simulink model "non_linear_sys_2"  (R2021b)
settings: Solver=FixedStepAuto  StartTime=0.0  StopTime=tfinal  FixedStep=dt  RelTol=1e-3
values from neighbouring files (symbols this model uses):
  dt = 1e-3    (= 0.001)    [data.m]
  g = 9.81    [data.m]
  IC = [0.0 0.0]    [data.m]    (also in postproc2.m)
  Jb = 2/5 * mb * rb^2    (= 4.24e-05)    [data.m]
  Lx = 0.143    [data.m]    (also in robust.m = Rx*M*Gx)
  Ly = 0.184    [data.m]    (also in robust.m = Rx*M*Gy)
  mb = 0.265    [data.m]    (also in robust.m = ureal('mb',mb,'Percentage',50))
  PID_sim = PID(PID_idx(ii))    [postproc2.m]
  rb = 0.02    [data.m]    (also in robust.m = ureal('rb',rb,'Percentage',20))
  rm = 0.025    [data.m]
undefined symbols (not defined in the file or in its folder): ref
libraries: simulink x6, slpidlib x2
settings Model: Creator=Daniele Oranges  LastModifiedBy=Daniele Oranges

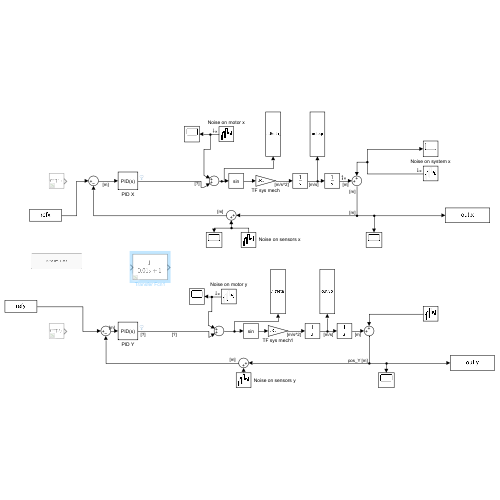
[thumbnail: Simulink's stored preview of the top-level diagram]
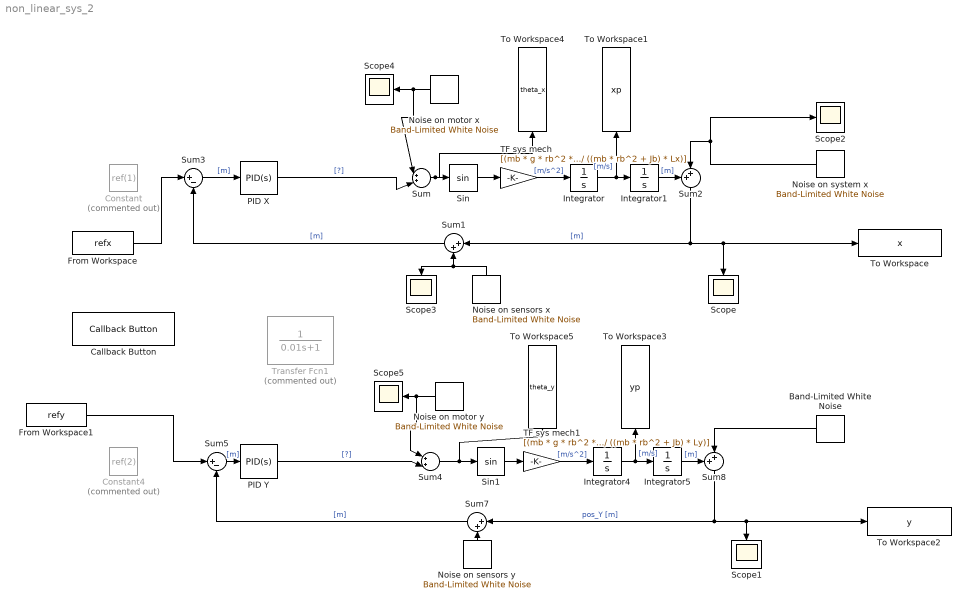
== system non_linear_sys_2 ==
  Band-Limited White Noise : simulink/Sources/Band-Limited White Noise  Cov=N.system  Ts=dt  seed=[23341]
  Callback Button : CallbackButton  ButtonText=Initialize Data
      settings: ClickFcn=|
      | clear
      | data
  Constant : Constant  Commented=on  Value=ref(1)
  Constant4 : Constant  Commented=on  Value=ref(2)
  From Workspace : FromWorkspace  VariableName=refx
  From Workspace1 : FromWorkspace  VariableName=refy
  Integrator : Integrator  InitialCondition=IC.velocity(1)
  Integrator1 : Integrator  InitialCondition=IC.position(1)
  Integrator4 : Integrator  InitialCondition=IC.velocity(2)
  Integrator5 : Integrator  InitialCondition=IC.position(2)
  Noise on motor x : simulink/Sources/Band-Limited White Noise  Cov=N.tension  Ts=dt  seed=[23341]
  Noise on motor y : simulink/Sources/Band-Limited White Noise  Cov=N.tension  Ts=dt  seed=[23341]
  Noise on sensors x : simulink/Sources/Band-Limited White Noise  Cov=N.sensor  Ts=dt  seed=[23341]
  Noise on sensors y : simulink/Sources/Band-Limited White Noise  Cov=N.sensor  Ts=dt  seed=[23341]
  Noise on system x : simulink/Sources/Band-Limited White Noise  Cov=N.system  Ts=dt  seed=[23341]
  PID X : slpidlib/PID Controller  Controller=PID  Form=Parallel  TimeDomain=Continuous-time  UseExternalTs=off  SampleTime=-1  IntegratorMethod=Forward Euler  FilterMethod=Forward Euler  ControllerParametersSource=internal  P=PID_sim.Kp  I=PID_sim.Ki  D=PID_sim.Kd  UseFilter=on  N=PID_sim.filter  TunerSelectOption=Transfer Function Based (PID Tuner App)  InitialConditionSource=internal  InitialConditionForIntegrator=0  InitialConditionForFilter=0  DifferentiatorICPrevScaledInput=0  ExternalReset=none  TrackingMode=off  Kt=1  LimitOutput=off  SatLimitsSource=internal  UpperSaturationLimit=inf  LowerSaturationLimit=-inf  LinearizeAsGain=on  AntiWindupMode=none  Kb=1  POutMin=[]  POutMax=[]  IOutMin=[]  IOutMax=[]  DOutMin=[]  DOutMax=[]  NOutMin=[]  NOutMax=[]  SumOutMin=[]  SumOutMax=[]  SaturationOutMin=[]  SaturationOutMax=[]  PParamMin=[]  PParamMax=[]  IParamMin=[]  IParamMax=[]  DParamMin=[]  DParamMax=[]  NParamMin=[]  NParamMax=[]  KbParamMin=[]  KbParamMax=[]  KtParamMin=[]  KtParamMax=[]  KbOutMin=[]  KbOutMax=[]  KtOutMin=[]  KtOutMax=[]  IntegratorOutMin=[]  IntegratorOutMax=[]  FilterOutMin=[]  FilterOutMax=[]  SumI1OutMin=[]  SumI1OutMax=[]  SumI2OutMin=[]  SumI2OutMax=[]  SumI3OutMin=[]  SumI3OutMax=[]  SumI4OutMin=[]  SumI4OutMax=[]  SumDOutMin=[]  SumDOutMax=[]  DifferentiatorOutMin=[]  DifferentiatorOutMax=[]  FilterDiffOutCoefMin=[]  FilterDiffOutCoefMax=[]  ReciprocalOutMin=[]  ReciprocalOutMax=[]  SumDenOutMin=[]  SumDenOutMax=[]  SumNumOutMin=[]  SumNumOutMax=[]  DivideOutMin=[]  DivideOutMax=[]  UdiffTsProdOutMin=[]  UdiffTsProdOutMax=[]  NTsProdOutMin=[]  NTsProdOutMax=[]  UintegralTsProdOutMin=[]  UintegralTsProdOutMax=[]  UngainTsProdOutMin=[]  UngainTsProdOutMax=[]  IntegratorContinuousStateAttributes=''  IntegratorStateMustResolveToSignalObject=off  IntegratorRTWStateStorageClass=Auto  FilterContinuousStateAttributes=''  FilterStateMustResolveToSignalObject=off  FilterRTWStateStorageClass=Auto  ParallelPVariant=InternalParameters  IdealPVariant=Disabled  IVariant=InternalParameters  DVariant=InternalParameters  IntegratorVariant=Continuous  SatVariant=Disabled  AWVariant=Passthrough  PCopyVariant=Disabled  TRVariant=Disabled  FdbkBlocksVariant=Forward  IdealPFdbkVariant=Disabled  SatFdbkVariant=Disabled  DerivativeFilterVariant=ContFilter  NVariant=InternalParameters  NCopyVariant=Disabled  FilterICVariant=InternalICsFilter  IntegratorICVariant=InternalICs  ExternalResetVariant=Disabled  TRSumVariant=Passthrough  SumFdbkVariant=Disabled  SumVariant=Sum_PID  TsampFilterVariant=InternalTs  TsampNgainVariant=Passthrough  TsampIntegralVariant=Passthrough  ExternalSaturationOutDataTypeStr=Inherit: Same as second input
  PID Y : slpidlib/PID Controller  Controller=PID  Form=Parallel  TimeDomain=Continuous-time  UseExternalTs=off  SampleTime=-1  IntegratorMethod=Forward Euler  FilterMethod=Forward Euler  ControllerParametersSource=internal  P=PID_sim.Kp  I=PID_sim.Ki  D=PID_sim.Kd  UseFilter=on  N=PID_sim.filter  TunerSelectOption=Transfer Function Based (PID Tuner App)  InitialConditionSource=internal  InitialConditionForIntegrator=0  InitialConditionForFilter=0  DifferentiatorICPrevScaledInput=0  ExternalReset=none  TrackingMode=off  Kt=1  LimitOutput=off  SatLimitsSource=internal  UpperSaturationLimit=inf  LowerSaturationLimit=-inf  LinearizeAsGain=on  AntiWindupMode=none  Kb=1  POutMin=[]  POutMax=[]  IOutMin=[]  IOutMax=[]  DOutMin=[]  DOutMax=[]  NOutMin=[]  NOutMax=[]  SumOutMin=[]  SumOutMax=[]  SaturationOutMin=[]  SaturationOutMax=[]  PParamMin=[]  PParamMax=[]  IParamMin=[]  IParamMax=[]  DParamMin=[]  DParamMax=[]  NParamMin=[]  NParamMax=[]  KbParamMin=[]  KbParamMax=[]  KtParamMin=[]  KtParamMax=[]  KbOutMin=[]  KbOutMax=[]  KtOutMin=[]  KtOutMax=[]  IntegratorOutMin=[]  IntegratorOutMax=[]  FilterOutMin=[]  FilterOutMax=[]  SumI1OutMin=[]  SumI1OutMax=[]  SumI2OutMin=[]  SumI2OutMax=[]  SumI3OutMin=[]  SumI3OutMax=[]  SumI4OutMin=[]  SumI4OutMax=[]  SumDOutMin=[]  SumDOutMax=[]  DifferentiatorOutMin=[]  DifferentiatorOutMax=[]  FilterDiffOutCoefMin=[]  FilterDiffOutCoefMax=[]  ReciprocalOutMin=[]  ReciprocalOutMax=[]  SumDenOutMin=[]  SumDenOutMax=[]  SumNumOutMin=[]  SumNumOutMax=[]  DivideOutMin=[]  DivideOutMax=[]  UdiffTsProdOutMin=[]  UdiffTsProdOutMax=[]  NTsProdOutMin=[]  NTsProdOutMax=[]  UintegralTsProdOutMin=[]  UintegralTsProdOutMax=[]  UngainTsProdOutMin=[]  UngainTsProdOutMax=[]  IntegratorContinuousStateAttributes=''  IntegratorStateMustResolveToSignalObject=off  IntegratorRTWStateStorageClass=Auto  FilterContinuousStateAttributes=''  FilterStateMustResolveToSignalObject=off  FilterRTWStateStorageClass=Auto  ParallelPVariant=InternalParameters  IdealPVariant=Disabled  IVariant=InternalParameters  DVariant=InternalParameters  IntegratorVariant=Continuous  SatVariant=Disabled  AWVariant=Passthrough  PCopyVariant=Disabled  TRVariant=Disabled  FdbkBlocksVariant=Forward  IdealPFdbkVariant=Disabled  SatFdbkVariant=Disabled  DerivativeFilterVariant=ContFilter  NVariant=InternalParameters  NCopyVariant=Disabled  FilterICVariant=InternalICsFilter  IntegratorICVariant=InternalICs  ExternalResetVariant=Disabled  TRSumVariant=Passthrough  SumFdbkVariant=Disabled  SumVariant=Sum_PID  TsampFilterVariant=InternalTs  TsampNgainVariant=Passthrough  TsampIntegralVariant=Passthrough  ExternalSaturationOutDataTypeStr=Inherit: Same as second input
  Scope{,1..5} (6 alike) : Scope
  Sin : Trigonometry
  Sin1 : Trigonometry
  Sum : Sum  Inputs=|++|
  Sum1 : Sum  Inputs=|++
  Sum2 : Sum  Inputs=++|
  Sum3 : Sum  Inputs=|+-
  Sum4 : Sum  Inputs=|++|
  Sum5 : Sum  Inputs=|+-
  Sum7 : Sum  Inputs=|++
  Sum8 : Sum  Inputs=++|
  TF sys mech : Gain  Gain=[(mb * g * rb^2 * rm * 10) / ((mb * rb^2 + Jb) * Lx)]
  TF sys mech1 : Gain  Gain=[(mb * g * rb^2 * rm) / ((mb * rb^2 + Jb) * Ly)]
  To Workspace : ToWorkspace  VariableName=x  SaveFormat=Timeseries  SampleTime=-1
  To Workspace1 : ToWorkspace  VariableName=xp  SaveFormat=Timeseries  SampleTime=-1
  To Workspace2 : ToWorkspace  VariableName=y  SaveFormat=Timeseries  SampleTime=-1
  To Workspace3 : ToWorkspace  VariableName=yp  SaveFormat=Timeseries  SampleTime=-1
  To Workspace4 : ToWorkspace  VariableName=theta_x  SaveFormat=Timeseries  SampleTime=-1
  To Workspace5 : ToWorkspace  VariableName=theta_y  SaveFormat=Timeseries  SampleTime=-1
  Transfer Fcn1 : TransferFcn  Commented=on  Denominator=[0.01 1]
  wires:
  Sum3/1 -> PID X/1  "[m]"
  Integrator/1 -> To Workspace1/1, Integrator1/1  "[m/s]"
  TF sys mech/1 -> Integrator/1  "[m/s^2]"
  Sin/1 -> TF sys mech/1
  TF sys mech1/1 -> Integrator4/1  "[m/s^2]"
  Sin1/1 -> TF sys mech1/1
  Sum5/1 -> PID Y/1  "[m]"
  PID Y/1 -> Sum4/2  "[?]"
  Sum8/1 -> Sum7/1, To Workspace2/1, Scope1/1  "pos_Y [m]"
  Integrator4/1 -> To Workspace3/1, Integrator5/1  "[m/s]"
  Noise on sensors x/1 -> Scope3/1, Sum1/2
  Sum1/1 -> Sum3/2  "[m]"
  Sum2/1 -> To Workspace/1, Scope/1, Sum1/1  "[m]"
  Integrator1/1 -> Sum2/1  "[m]"
  Noise on system x/1 -> Scope2/1, Sum2/2
  Sum7/1 -> Sum5/2  "[m]"
  Noise on sensors y/1 -> Sum7/2
  Integrator5/1 -> Sum8/1  "[m]"
  Band-Limited White Noise/1 -> Sum8/2
  Sum/1 -> To Workspace4/1, Sin/1
  Noise on motor x/1 -> Sum/1, Scope4/1
  PID X/1 -> Sum/2  "[?]"
  Sum4/1 -> To Workspace5/1, Sin1/1
  Noise on motor y/1 -> Sum4/1, Scope5/1
  From Workspace/1 -> Sum3/1
  From Workspace1/1 -> Sum5/1
